simulink model "modelo_matematico"  (R2018b)
settings: Solver=ode4  StartTime=0.0  StopTime=t_f  FixedStep=fst  RelTol=1e-3  EnableMultiTasking=on
values from neighbouring files (symbols this model uses):
  a = plot(dado_t, dado_vd, '-', 'Color',[1.0,0.5,0.0], 'LineWidth', 4)    [Graficos.m]    (also in Trajetoria_OITO_8.m = 0.09)
  b = plot(dado_t, dado_vr, '-', 'Color',[0.0,0.0,0.0], 'LineWidth', 1)    [Graficos.m]    (also in Script_principal.m = 0.121)
  c_d = r_d/(2*b)    (= 0.120661157025)    [Script_principal.m]
  c_e = r_e/(2*b)    (= 0.121074380165)    [Script_principal.m]
  fD = 0.0069    [Script_principal.m]
  fD_v = var_fD*0.0069    (= 0.0069)    [Script_principal.m]
  fE = 0.0053    [Script_principal.m]
  fE_v = var_fE*0.0053    (= 0.0053)    [Script_principal.m]
  fst = 0.001    [Script_principal.m]
  I = 0.0903    [Script_principal.m]
  I_v = var_I*0.0903    (= 0.0903)    [Script_principal.m]
  Ir = 0.00094    [Script_principal.m]
  Ir_v = var_Ir*0.00094    (= 0.00094)    [Script_principal.m]
  k0 = 25    [Script_principal.m]
  k1 = 25    [Script_principal.m]
  KaD = 0.4713    [Script_principal.m]
  KaD_v = var_KaD*0.4713    (= 0.4713)    [Script_principal.m]
  KaE = 0.5046    [Script_principal.m]
  KaE_v = var_KaE*0.5046    (= 0.5046)    [Script_principal.m]
  KtD = KaD    (= 0.4713)    [Script_principal.m]
  KtD_v = var_KtD*KaD    (= 0.4713)    [Script_principal.m]
  KtE = KaE    (= 0.5046)    [Script_principal.m]
  KtE_v = var_KtE*KaE    (= 0.5046)    [Script_principal.m]
  L = 0.10    (= 0.1)    [Script_principal.m]
  m = 1.932    [Script_principal.m]
  m_v = var_m*1.932    (= 1.932)    [Script_principal.m]
  NL = 0    [Script_principal.m]
  npD = 0.0001    [Script_principal.m]
  npE = 0.0001    [Script_principal.m]
  r_d = 0.0292    [Script_principal.m]
  r_e = 0.0293    [Script_principal.m]
  RaD = 8.4507    [Script_principal.m]
  RaD_v = var_RaD*8.4507    (= 8.4507)    [Script_principal.m]
  RaE = 7.7177    [Script_principal.m]
  RaE_v = var_RaE*7.7177    (= 7.7177)    [Script_principal.m]
  T = 4    [Script_principal.m]
  t_f = t_i+dur_r+dur_8+dur_r    [Trajetoria_OITO_8.m]
  t_i = 0    [Trajetoria_OITO_8.m]
  t_i_1 = t_i+dur_r    (= 3.33333333333)    [Trajetoria_OITO_8.m]
  t_i_2 = t_i+dur_r+dur_8    [Trajetoria_OITO_8.m]
  v = 0.30    (= 0.3)    [Trajetoria_OITO_8.m]
  VaD_max = 14    [Script_principal.m]
  VaE_max = 14    [Script_principal.m]
  vel_ang_D = 4    [Script_principal.m]
  vel_ang_E = 4    [Script_principal.m]
  wx = v/raio_x    (= 0.3)    [Trajetoria_OITO_8.m]
  wy = v/raio_y    (= 0.6)    [Trajetoria_OITO_8.m]
  x0 = [x0_1; x0_2; x0_3; x0_4; x0_5; x0_6]    [Script_principal.m]
undefined symbols (not defined in the file or in its folder): dur_c, t_i_3, t_i_c, time_c, w
libraries: simulink x41, dspmtrx3 x8
settings Model: Creator=nenem  LastModifiedBy=nenem
settings OptimizationCC: LifeSpan=inf
settings DebuggingCC: SFUnexpectedBacktrackingDiag=warning  SFNoUnconditionalDefaultTransitionDiag=warning
settings SFSimCC: SimUseLocalCustomCode=off
settings RTWCC: RTWUseLocalCustomCode=off
settings CodeAppCC: StateflowObjectComments=on
settings GRTTargetCC: TargetLangStandard=C89/C90 (ANSI)  GeneratePreprocessorConditionals=Disable all
settings ConfigComp: CovMetricSettings=dw  CovHtmlReporting=on  CovSaveCumulativeToWorkspaceVar=on  CovSaveSingleToWorkspaceVar=on  CovExternalEMLEnable=off

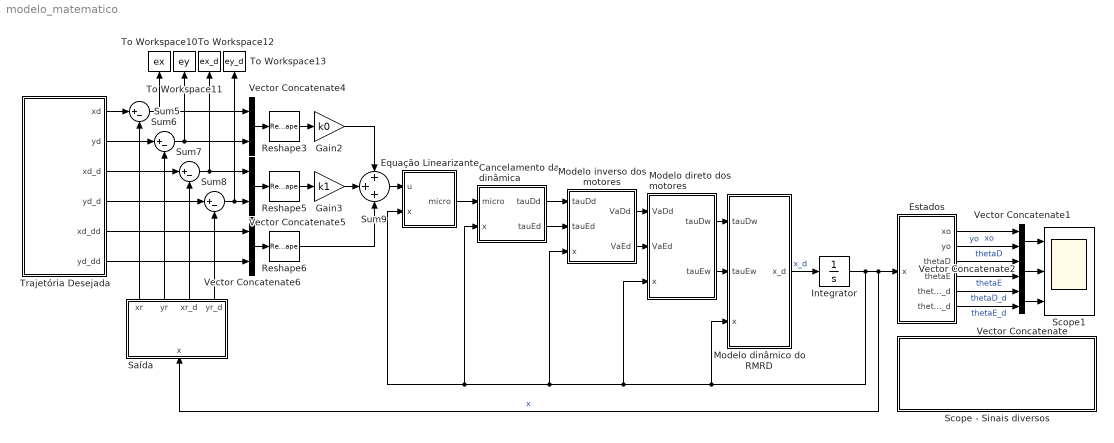
== system modelo_matematico ==
  Cancelamento da dinâmica : Subsystem
  Equação Linearizante : Subsystem
  Estados : Subsystem
  Gain2 : Gain  Gain=k0
  Gain3 : Gain  Gain=k1
  Integrator : Integrator  InitialCondition=x0
  Modelo dinâmico do RMRD : Subsystem
  Modelo direto dos motores : Subsystem
  Modelo inverso dos motores : Subsystem
  Reshape3 : Reshape  OutputDimensionality=Customize  OutputDimensions=[2,1]
  Reshape5 : Reshape  OutputDimensionality=Customize  OutputDimensions=[2,1]
  Reshape6 : Reshape  OutputDimensionality=Customize  OutputDimensions=[2,1]
  Saída : Subsystem
  Scope - Sinais diversos : Subsystem
  Scope1 : Scope  NumInputPorts=3
  Sum{5..8} (4 alike) : Sum  Inputs=|+-
  Sum9 : Sum  Inputs=+++
  To Workspace10 : ToWorkspace  VariableName=ex  SaveFormat=Structure With Time  SampleTime=-1
      settings: Save2DSignal=2-D array (concatenate along first dimension)
  To Workspace11 : ToWorkspace  VariableName=ey  SaveFormat=Structure With Time  SampleTime=-1
      settings: Save2DSignal=2-D array (concatenate along first dimension)
  To Workspace12 : ToWorkspace  VariableName=ex_d  SaveFormat=Structure With Time  SampleTime=-1
      settings: Save2DSignal=2-D array (concatenate along first dimension)
  To Workspace13 : ToWorkspace  VariableName=ey_d  SaveFormat=Structure With Time  SampleTime=-1
      settings: Save2DSignal=2-D array (concatenate along first dimension)
  Trajetória Desejada : Subsystem
  Vector Concatenate{,1..2,4..6} (6 alike) : Concatenate
  wires:
  Reshape6/1 -> Sum9/3
  Vector Concatenate6/1 -> Reshape6/1
  Reshape5/1 -> Gain3/1
  Sum7/1 -> Vector Concatenate5/1, To Workspace12/1
  Gain2/1 -> Sum9/1
  Equação Linearizante/1(micro) -> Cancelamento da dinâmica/1(micro)
  Sum8/1 -> Vector Concatenate5/2, To Workspace13/1
  Sum9/1 -> Equação Linearizante/1(u)
  Reshape3/1 -> Gain2/1
  Vector Concatenate5/1 -> Reshape5/1
  Vector Concatenate4/1 -> Reshape3/1
  Trajetória Desejada/3(xd_d) -> Sum7/1
  Trajetória Desejada/5(xd_dd) -> Vector Concatenate6/1
  Gain3/1 -> Sum9/2
  Trajetória Desejada/4(yd_d) -> Sum8/1
  Trajetória Desejada/2(yd) -> Sum6/1
  Trajetória Desejada/1(xd) -> Sum5/1
  Modelo dinâmico do RMRD/1(x_d) -> Integrator/1  "x_d"
  Integrator/1 -> Saída/1(x), Estados/1(x), Equação Linearizante/2(x), Cancelamento da dinâmica/2(x), Modelo inverso dos motores/3(x), Modelo direto dos motores/3(x), Modelo dinâmico do RMRD/3(x)  "x"
  Cancelamento da dinâmica/1(tauDd) -> Modelo inverso dos motores/1(tauDd)
  Cancelamento da dinâmica/2(tauEd) -> Modelo inverso dos motores/2(tauEd)
  Modelo direto dos motores/1(tauDw) -> Modelo dinâmico do RMRD/1(tauDw)
  Modelo direto dos motores/2(tauEw) -> Modelo dinâmico do RMRD/2(tauEw)
  Modelo inverso dos motores/2(VaEd) -> Modelo direto dos motores/2(VaEd)
  Modelo inverso dos motores/1(VaDd) -> Modelo direto dos motores/1(VaDd)
  Saída/1(xr) -> Sum5/2
  Saída/2(yr) -> Sum6/2
  Saída/3(xr_d) -> Sum7/2
  Saída/4(yr_d) -> Sum8/2
  Vector Concatenate1/1 -> Scope1/1
  Vector Concatenate2/1 -> Scope1/2
  Vector Concatenate/1 -> Scope1/3
  Estados/4(thetaE) -> Vector Concatenate2/2  "thetaE"
  Estados/1(xo) -> Vector Concatenate1/1  "xo"
  Estados/3(thetaD) -> Vector Concatenate2/1  "thetaD"
  Estados/2(yo) -> Vector Concatenate1/2  "yo"
  Estados/5(thetaD_d) -> Vector Concatenate/1  "thetaD_d"
  Estados/6(thetaE_d) -> Vector Concatenate/2  "thetaE_d"
  Trajetória Desejada/6(yd_dd) -> Vector Concatenate6/2
  Sum5/1 -> Vector Concatenate4/1, To Workspace10/1
  Sum6/1 -> Vector Concatenate4/2, To Workspace11/1

== system modelo_matematico/Cancelamento da dinâmica ==
  micro : Inport
  x : Inport  Port=2
  Constant1 : Constant  Value=[b r_d r_e c_d c_e Ir_v m_v I_v]
  Reshape7 : Reshape  OutputDimensionality=Customize  OutputDimensions=[1,8]
  To Workspace18 : ToWorkspace  VariableName=tauDd  SaveFormat=Structure With Time  SampleTime=-1
      settings: Save2DSignal=2-D array (concatenate along first dimension)
  To Workspace19 : ToWorkspace  VariableName=tauEd  SaveFormat=Structure With Time  SampleTime=-1
      settings: Save2DSignal=2-D array (concatenate along first dimension)
  Transformação da Entrada : MATLAB Function  TreatAsAtomicUnit=on
  tauDd : Outport
  tauEd : Outport  Port=2
  tag scope: tauDd=global, tauEd=global
  wires:
  micro/1 -> Transformação da Entrada/2(micro)
  Constant1/1 -> Reshape7/1
  Reshape7/1 -> Transformação da Entrada/1(cte)
  x/1 -> Transformação da Entrada/3(x)
  Transformação da Entrada/2(tauE) -> tauEd/1, To Workspace19/1, [tauEd]
  Transformação da Entrada/1(tauD) -> tauDd/1, To Workspace18/1, [tauDd]

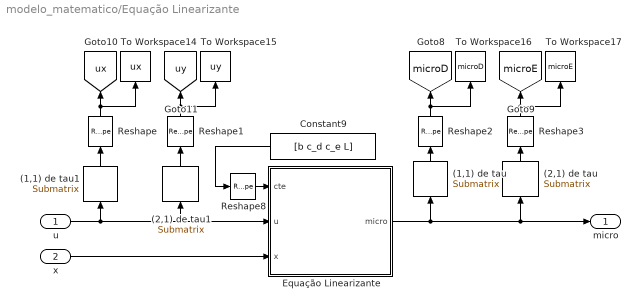
== system modelo_matematico/Equação Linearizante ==
  u : Inport
  x : Inport  Port=2
  (1,1) de tau : dspmtrx3/Submatrix  RowSpan=One row  RowStartMode=Index  RowStartIndex=1  RowEndMode=Last  RowEndIndex=1  ColSpan=One column  ColStartMode=Index  ColStartIndex=1  ColEndMode=Last  ColEndIndex=1
  (1,1) de tau1 : dspmtrx3/Submatrix  RowSpan=One row  RowStartMode=Index  RowStartIndex=1  RowEndMode=Last  RowEndIndex=1  ColSpan=One column  ColStartMode=Index  ColStartIndex=1  ColEndMode=Last  ColEndIndex=1
  (2,1) de tau : dspmtrx3/Submatrix  RowSpan=One row  RowStartMode=Index  RowStartIndex=2  RowEndMode=Last  RowEndIndex=1  ColSpan=One column  ColStartMode=Index  ColStartIndex=1  ColEndMode=Last  ColEndIndex=1
  (2,1) de tau1 : dspmtrx3/Submatrix  RowSpan=One row  RowStartMode=Index  RowStartIndex=2  RowEndMode=Last  RowEndIndex=1  ColSpan=One column  ColStartMode=Index  ColStartIndex=1  ColEndMode=Last  ColEndIndex=1
  Constant9 : Constant  Value=[b c_d c_e L]
  Equação Linearizante : MATLAB Function  TreatAsAtomicUnit=on
  Reshape{,1..3} (4 alike) : Reshape
  Reshape8 : Reshape  OutputDimensionality=Customize  OutputDimensions=[1,4]
  To Workspace14 : ToWorkspace  VariableName=ux  SaveFormat=Structure With Time  SampleTime=-1
      settings: Save2DSignal=2-D array (concatenate along first dimension)
  To Workspace15 : ToWorkspace  VariableName=uy  SaveFormat=Structure With Time  SampleTime=-1
      settings: Save2DSignal=2-D array (concatenate along first dimension)
  To Workspace16 : ToWorkspace  VariableName=microD  SaveFormat=Structure With Time  SampleTime=-1
      settings: Save2DSignal=2-D array (concatenate along first dimension)
  To Workspace17 : ToWorkspace  VariableName=microE  SaveFormat=Structure With Time  SampleTime=-1
      settings: Save2DSignal=2-D array (concatenate along first dimension)
  micro : Outport
  tag scope: microD=global, microE=global, ux=global, uy=global
  wires:
  Constant9/1 -> Reshape8/1
  Reshape8/1 -> Equação Linearizante/1(cte)
  x/1 -> Equação Linearizante/3(x)
  (2,1) de tau1/1 -> Reshape1/1
  (1,1) de tau1/1 -> Reshape/1
  u/1 -> (1,1) de tau1/1, (2,1) de tau1/1, Equação Linearizante/2(u)
  Reshape/1 -> To Workspace14/1, [ux]
  Reshape1/1 -> To Workspace15/1, [uy]
  Reshape3/1 -> To Workspace17/1, [microE]
  Reshape2/1 -> To Workspace16/1, [microD]
  (2,1) de tau/1 -> Reshape3/1
  Equação Linearizante/1(micro) -> micro/1, (2,1) de tau/1, (1,1) de tau/1
  (1,1) de tau/1 -> Reshape2/1

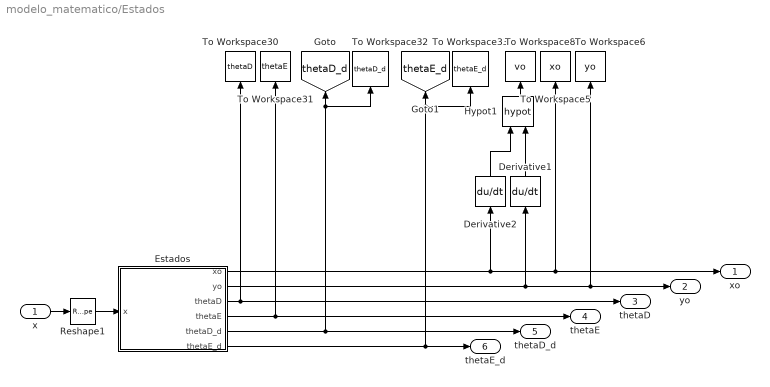
== system modelo_matematico/Estados ==
  x : Inport
  Derivative1 : Derivative
  Derivative2 : Derivative
  Estados : MATLAB Function  TreatAsAtomicUnit=on
  Hypot1 : Math  Operator=hypot  SaturateOnIntegerOverflow=on
  Reshape1 : Reshape  OutputDimensionality=Customize  OutputDimensions=[6,1]
  To Workspace30 : ToWorkspace  VariableName=thetaD  SaveFormat=Structure With Time  SampleTime=-1
      settings: Save2DSignal=2-D array (concatenate along first dimension)
  To Workspace31 : ToWorkspace  VariableName=thetaE  SaveFormat=Structure With Time  SampleTime=-1
      settings: Save2DSignal=2-D array (concatenate along first dimension)
  To Workspace32 : ToWorkspace  VariableName=thetaD_d  SaveFormat=Structure With Time  SampleTime=-1
      settings: Save2DSignal=2-D array (concatenate along first dimension)
  To Workspace33 : ToWorkspace  VariableName=thetaE_d  SaveFormat=Structure With Time  SampleTime=-1
      settings: Save2DSignal=2-D array (concatenate along first dimension)
  To Workspace5 : ToWorkspace  VariableName=xo  SaveFormat=Structure With Time  SampleTime=-1
      settings: Save2DSignal=2-D array (concatenate along first dimension)
  To Workspace6 : ToWorkspace  VariableName=yo  SaveFormat=Structure With Time  SampleTime=-1
      settings: Save2DSignal=2-D array (concatenate along first dimension)
  To Workspace8 : ToWorkspace  VariableName=vo  SaveFormat=Structure With Time  SampleTime=-1
      settings: Save2DSignal=2-D array (concatenate along first dimension)
  xo : Outport
  yo : Outport  Port=2
  thetaD : Outport  Port=3
  thetaE : Outport  Port=4
  thetaD_d : Outport  Port=5
  thetaE_d : Outport  Port=6
  tag scope: thetaD_d=global, thetaE_d=global
  wires:
  x/1 -> Reshape1/1
  Estados/5(thetaD_d) -> thetaD_d/1, To Workspace32/1, [thetaD_d]
  Estados/6(thetaE_d) -> thetaE_d/1, To Workspace33/1, [thetaE_d]
  Estados/1(xo) -> xo/1, To Workspace5/1, Derivative2/1
  Derivative2/1 -> Hypot1/1
  Estados/2(yo) -> yo/1, To Workspace6/1, Derivative1/1
  Derivative1/1 -> Hypot1/2
  Hypot1/1 -> To Workspace8/1
  Estados/3(thetaD) -> thetaD/1, To Workspace30/1
  Estados/4(thetaE) -> thetaE/1, To Workspace31/1
  Reshape1/1 -> Estados/1(x)

== system modelo_matematico/Modelo dinâmico do RMRD ==
  tauDw : Inport
  tauEw : Inport  Port=2
  x : Inport  Port=3
  Constant1 : Constant  Value=[b r_d r_e c_d c_e Ir m I]
  Manual Switch : ManualSwitch
  Modelo do WMR : MATLAB Function  TreatAsAtomicUnit=on
  Não idealidades : Subsystem  Commented=on
  Reshape2 : Reshape  OutputDimensionality=Customize  OutputDimensions=[1,8]
  Reshape3 : Reshape  OutputDimensionality=Customize  OutputDimensions=[6,1]
  x_d : Outport
  wires:
  tauEw/1 -> Modelo do WMR/3(tau_E)
  tauDw/1 -> Modelo do WMR/2(tau_D)
  Reshape2/1 -> Modelo do WMR/1(cte)
  Modelo do WMR/1(x_d) -> Reshape3/1  "x_d"
  x/1 -> Modelo do WMR/4(x)
  Reshape3/1 -> Manual Switch/1, Não idealidades/1(In)
  Manual Switch/1 -> x_d/1
  Constant1/1 -> Reshape2/1
  Não idealidades/1(Out) -> Manual Switch/2

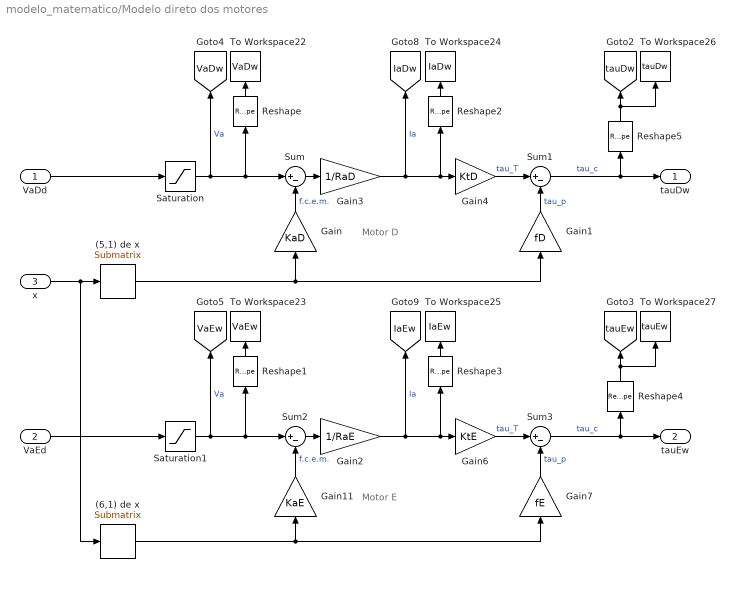
== system modelo_matematico/Modelo direto dos motores ==
  note: Motor D
  note: Motor E
  VaDd : Inport
  VaEd : Inport  Port=2
  x : Inport  Port=3
  (5,1) de x : dspmtrx3/Submatrix  RowSpan=One row  RowStartMode=Index  RowStartIndex=5  RowEndMode=Last  RowEndIndex=1  ColSpan=One column  ColStartMode=Index  ColStartIndex=1  ColEndMode=Last  ColEndIndex=1
  (6,1) de x : dspmtrx3/Submatrix  RowSpan=One row  RowStartMode=Index  RowStartIndex=6  RowEndMode=Last  RowEndIndex=1  ColSpan=One column  ColStartMode=Index  ColStartIndex=1  ColEndMode=Last  ColEndIndex=1
  Gain : Gain  Gain=KaD
  Gain1 : Gain  Gain=fD
  Gain11 : Gain  Gain=KaE
  Gain2 : Gain  Gain=1/RaE
  Gain3 : Gain  Gain=1/RaD
  Gain4 : Gain  Gain=KtD
  Gain6 : Gain  Gain=KtE
  Gain7 : Gain  Gain=fE
  Reshape{,1..5} (6 alike) : Reshape
  Saturation : Saturate  UpperLimit=VaD_max  LowerLimit=-VaD_max
  Saturation1 : Saturate  UpperLimit=VaE_max  LowerLimit=-VaE_max
  Sum{,1..3} (4 alike) : Sum  Inputs=|+-
  To Workspace22 : ToWorkspace  VariableName=VaDw  SaveFormat=Structure With Time  SampleTime=-1
      settings: Save2DSignal=2-D array (concatenate along first dimension)
  To Workspace23 : ToWorkspace  VariableName=VaEw  SaveFormat=Structure With Time  SampleTime=-1
      settings: Save2DSignal=2-D array (concatenate along first dimension)
  To Workspace24 : ToWorkspace  VariableName=IaDw  SaveFormat=Structure With Time  SampleTime=-1
      settings: Save2DSignal=2-D array (concatenate along first dimension)
  To Workspace25 : ToWorkspace  VariableName=IaEw  SaveFormat=Structure With Time  SampleTime=-1
      settings: Save2DSignal=2-D array (concatenate along first dimension)
  To Workspace26 : ToWorkspace  VariableName=tauDw  SaveFormat=Structure With Time  SampleTime=-1
      settings: Save2DSignal=2-D array (concatenate along first dimension)
  To Workspace27 : ToWorkspace  VariableName=tauEw  SaveFormat=Structure With Time  SampleTime=-1
      settings: Save2DSignal=2-D array (concatenate along first dimension)
  tauDw : Outport
  tauEw : Outport  Port=2
  tag scope: IaDw=global, IaEw=global, VaDw=global, VaEw=global, tauDw=global, tauEw=global
  wires:
  Gain7/1 -> Sum3/2  "tau_p"
  Gain2/1 -> Reshape3/1, Gain6/1, [IaEw]  "Ia"
  (6,1) de x/1 -> Gain11/1, Gain7/1
  Gain6/1 -> Sum3/1  "tau_T"
  (5,1) de x/1 -> Gain1/1, Gain/1
  Gain11/1 -> Sum2/2  "f.c.e.m."
  Gain1/1 -> Sum1/2  "tau_p"
  Sum2/1 -> Gain2/1
  Gain4/1 -> Sum1/1  "tau_T"
  Gain/1 -> Sum/2  "f.c.e.m."
  Gain3/1 -> Reshape2/1, Gain4/1, [IaDw]  "Ia"
  Sum/1 -> Gain3/1
  Sum1/1 -> Reshape5/1, tauDw/1  "tau_c"
  Sum3/1 -> Reshape4/1, tauEw/1  "tau_c"
  x/1 -> (5,1) de x/1, (6,1) de x/1
  Saturation/1 -> [VaDw], Reshape/1, Sum/1  "Va"
  Saturation1/1 -> [VaEw], Reshape1/1, Sum2/1  "Va"
  Reshape/1 -> To Workspace22/1
  Reshape1/1 -> To Workspace23/1
  Reshape2/1 -> To Workspace24/1
  Reshape3/1 -> To Workspace25/1
  VaDd/1 -> Saturation/1
  VaEd/1 -> Saturation1/1
  Reshape4/1 -> To Workspace27/1, [tauEw]
  Reshape5/1 -> To Workspace26/1, [tauDw]

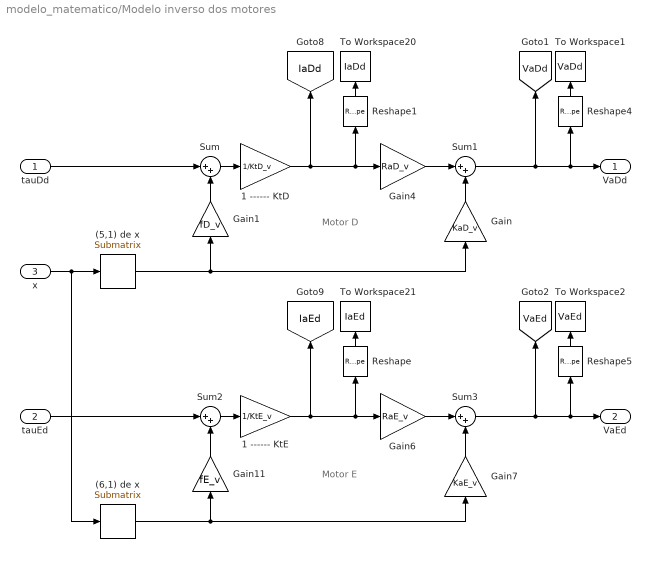
== system modelo_matematico/Modelo inverso dos motores ==
  note: Motor D
  note: Motor E
  tauDd : Inport
  tauEd : Inport  Port=2
  x : Inport  Port=3
  (5,1) de x : dspmtrx3/Submatrix  RowSpan=One row  RowStartMode=Index  RowStartIndex=5  RowEndMode=Last  RowEndIndex=1  ColSpan=One column  ColStartMode=Index  ColStartIndex=1  ColEndMode=Last  ColEndIndex=1
  (6,1) de x : dspmtrx3/Submatrix  RowSpan=One row  RowStartMode=Index  RowStartIndex=6  RowEndMode=Last  RowEndIndex=1  ColSpan=One column  ColStartMode=Index  ColStartIndex=1  ColEndMode=Last  ColEndIndex=1
  1 ------ KtD : Gain  Gain=1/KtD_v
  1 ------ KtE : Gain  Gain=1/KtE_v
  Gain : Gain  Gain=KaD_v
  Gain1 : Gain  Gain=fD_v
  Gain11 : Gain  Gain=fE_v
  Gain4 : Gain  Gain=RaD_v
  Gain6 : Gain  Gain=RaE_v
  Gain7 : Gain  Gain=KaE_v
  Reshape{,1,4..5} (4 alike) : Reshape
  Sum{,1..3} (4 alike) : Sum  Inputs=|++
  To Workspace1 : ToWorkspace  VariableName=VaDd  SaveFormat=Structure With Time  SampleTime=-1
      settings: Save2DSignal=2-D array (concatenate along first dimension)
  To Workspace2 : ToWorkspace  VariableName=VaEd  SaveFormat=Structure With Time  SampleTime=-1
      settings: Save2DSignal=2-D array (concatenate along first dimension)
  To Workspace20 : ToWorkspace  VariableName=IaDd  SaveFormat=Structure With Time  SampleTime=-1
      settings: Save2DSignal=2-D array (concatenate along first dimension)
  To Workspace21 : ToWorkspace  VariableName=IaEd  SaveFormat=Structure With Time  SampleTime=-1
      settings: Save2DSignal=2-D array (concatenate along first dimension)
  VaDd : Outport
  VaEd : Outport  Port=2
  tag scope: IaDd=global, IaEd=global, VaDd=global, VaEd=global
  wires:
  Gain7/1 -> Sum3/2
  1 ------ KtE/1 -> Reshape/1, Gain6/1, [IaEd]
  (6,1) de x/1 -> Gain11/1, Gain7/1
  Gain6/1 -> Sum3/1
  tauEd/1 -> Sum2/1
  (5,1) de x/1 -> Gain/1, Gain1/1
  Gain11/1 -> Sum2/2
  Gain/1 -> Sum1/2
  Sum2/1 -> 1 ------ KtE/1
  Gain4/1 -> Sum1/1
  Gain1/1 -> Sum/2
  1 ------ KtD/1 -> Reshape1/1, Gain4/1, [IaDd]
  Sum/1 -> 1 ------ KtD/1
  Sum1/1 -> [VaDd], VaDd/1, Reshape4/1
  Sum3/1 -> [VaEd], Reshape5/1, VaEd/1
  tauDd/1 -> Sum/1
  x/1 -> (6,1) de x/1, (5,1) de x/1
  Reshape/1 -> To Workspace21/1
  Reshape1/1 -> To Workspace20/1
  Reshape4/1 -> To Workspace1/1
  Reshape5/1 -> To Workspace2/1

== system modelo_matematico/Saída ==
  x : Inport
  Constant9 : Constant  Value=[b c_d c_e L]
  Hypot2 : Math  Operator=hypot  SaturateOnIntegerOverflow=on
  Reshape1 : Reshape  OutputDimensionality=Customize  OutputDimensions=[6,1]
  Reshape9 : Reshape  OutputDimensionality=Customize  OutputDimensions=[1,4]
  Saídas : MATLAB Function  TreatAsAtomicUnit=on
  To Workspace3 : ToWorkspace  VariableName=xr  SaveFormat=Structure With Time  SampleTime=-1
      settings: Save2DSignal=2-D array (concatenate along first dimension)
  To Workspace4 : ToWorkspace  VariableName=yr  SaveFormat=Structure With Time  SampleTime=-1
      settings: Save2DSignal=2-D array (concatenate along first dimension)
  To Workspace7 : ToWorkspace  VariableName=vr  SaveFormat=Structure With Time  SampleTime=-1
      settings: Save2DSignal=2-D array (concatenate along first dimension)
  xr : Outport
  yr : Outport  Port=2
  xr_d : Outport  Port=3
  yr_d : Outport  Port=4
  wires:
  Reshape9/1 -> Saídas/1(cte)
  Constant9/1 -> Reshape9/1
  x/1 -> Reshape1/1
  Saídas/3(xr_d) -> xr_d/1, Hypot2/1
  Saídas/4(yr_d) -> yr_d/1, Hypot2/2
  Saídas/1(xr) -> xr/1, To Workspace3/1
  Saídas/2(yr) -> yr/1, To Workspace4/1
  Hypot2/1 -> To Workspace7/1
  Reshape1/1 -> Saídas/2(x)

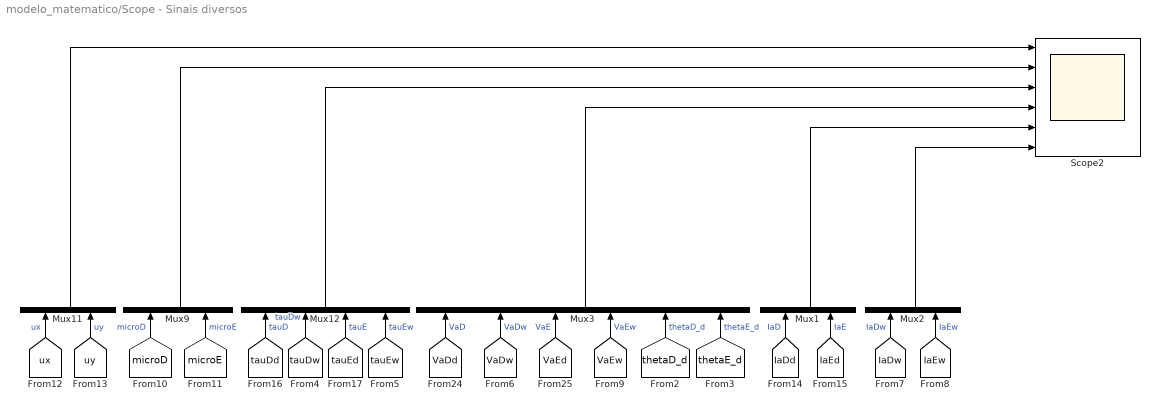
== system modelo_matematico/Scope - Sinais diversos ==
  Mux{1..2,9,11} (4 alike) : Mux  Inputs=2
  Mux12 : Mux
  Mux3 : Mux  Inputs=6
  Scope2 : Scope  NumInputPorts=6
  wires:
  [tauDd] -> Mux12/1  "tauD"
  [VaEw] -> Mux3/4  "VaEw"
  [IaEd] -> Mux1/2  "IaE"
  [ux] -> Mux11/1  "ux"
  [VaEd] -> Mux3/3  "VaE"
  [IaDd] -> Mux1/1  "IaD"
  [VaDw] -> Mux3/2  "VaDw"
  [tauEd] -> Mux12/3  "tauE"
  Mux12/1 -> Scope2/3
  [uy] -> Mux11/2  "uy"
  Mux3/1 -> Scope2/4
  [microD] -> Mux9/1  "microD"
  [microE] -> Mux9/2  "microE"
  [VaDd] -> Mux3/1  "VaD"
  Mux11/1 -> Scope2/1
  Mux9/1 -> Scope2/2
  Mux1/1 -> Scope2/5
  Mux2/1 -> Scope2/6
  [tauDw] -> Mux12/2  "tauDw"
  [tauEw] -> Mux12/4  "tauEw"
  [thetaD_d] -> Mux3/5  "thetaD_d"
  [thetaE_d] -> Mux3/6  "thetaE_d"
  [IaEw] -> Mux2/2  "IaEw"
  [IaDw] -> Mux2/1  "IaDw"

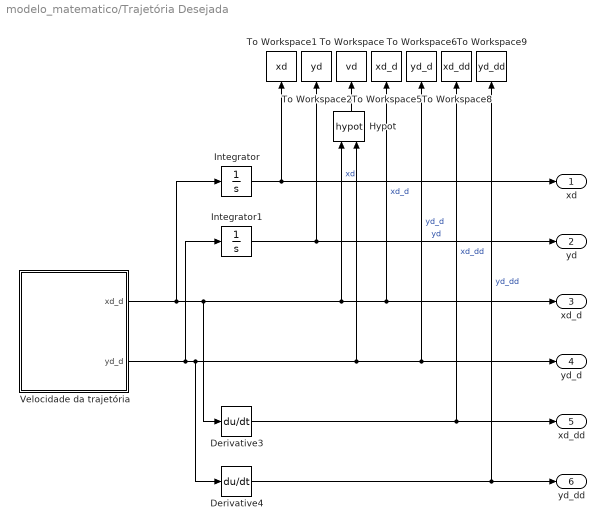
== system modelo_matematico/Trajetória Desejada ==
  Derivative3 : Derivative
  Derivative4 : Derivative
  Hypot : Math  Operator=hypot  OutputSignalType=real  SaturateOnIntegerOverflow=on
  Integrator : Integrator
  Integrator1 : Integrator
  To Workspace : ToWorkspace  VariableName=vd  SaveFormat=Structure With Time  SampleTime=-1
      settings: Save2DSignal=2-D array (concatenate along first dimension)
  To Workspace1 : ToWorkspace  VariableName=xd  SaveFormat=Structure With Time  SampleTime=-1
      settings: Save2DSignal=2-D array (concatenate along first dimension)
  To Workspace2 : ToWorkspace  VariableName=yd  SaveFormat=Structure With Time  SampleTime=-1
      settings: Save2DSignal=2-D array (concatenate along first dimension)
  To Workspace5 : ToWorkspace  VariableName=xd_d  SaveFormat=Structure With Time  SampleTime=-1
      settings: Save2DSignal=2-D array (concatenate along first dimension)
  To Workspace6 : ToWorkspace  VariableName=yd_d  SaveFormat=Structure With Time  SampleTime=-1
      settings: Save2DSignal=2-D array (concatenate along first dimension)
  To Workspace8 : ToWorkspace  VariableName=xd_dd  SaveFormat=Structure With Time  SampleTime=-1
      settings: Save2DSignal=2-D array (concatenate along first dimension)
  To Workspace9 : ToWorkspace  VariableName=yd_dd  SaveFormat=Structure With Time  SampleTime=-1
      settings: Save2DSignal=2-D array (concatenate along first dimension)
  Velocidade da trajetória : Subsystem
  xd : Outport
  yd : Outport  Port=2
  xd_d : Outport  Port=3
  yd_d : Outport  Port=4
  xd_dd : Outport  Port=5
  yd_dd : Outport  Port=6
  wires:
  Derivative3/1 -> xd_dd/1, To Workspace8/1  "xd_dd"
  Derivative4/1 -> yd_dd/1, To Workspace9/1  "yd_dd"
  Integrator/1 -> xd/1, To Workspace1/1  "xd"
  Integrator1/1 -> yd/1, To Workspace2/1  "yd"
  Hypot/1 -> To Workspace/1
  Velocidade da trajetória/1(xd_d) -> Integrator/1, Derivative3/1, xd_d/1, To Workspace5/1, Hypot/1  "xd_d"
  Velocidade da trajetória/2(yd_d) -> Integrator1/1, yd_d/1, To Workspace6/1, Hypot/2, Derivative4/1  "yd_d"

== system modelo_matematico/Modelo dinâmico do RMRD/Não idealidades ==
  In : Inport
  Não idealidades : Subsystem
  demux : MATLAB Function  TreatAsAtomicUnit=on
  mux : MATLAB Function  TreatAsAtomicUnit=on
  Out : Outport
  wires:
  In/1 -> demux/1(x)
  Não idealidades/1(OutD) -> mux/5(x5_d)
  Não idealidades/2(OutE) -> mux/6(x6_d)
  mux/1(x) -> Out/1
  demux/5(x5_d) -> Não idealidades/1(InD)
  demux/6(x6_d) -> Não idealidades/2(InE)
  demux/4(x4_d) -> mux/4(x4_d)
  demux/2(x2_d) -> mux/2(x2_d)
  demux/1(x1_d) -> mux/1(x1_d)
  demux/3(x3_d) -> mux/3(x3_d)

== system modelo_matematico/Trajetória Desejada/Velocidade da trajetória ==
  0 : Subsystem  Commented=on
  0 c/ RAMPA : Subsystem  Commented=on
  180 c/ RAMPA : Subsystem  Commented=on
  8 : Subsystem
  "90 " : Subsystem  Commented=on
  90 c/ RAMPA : Subsystem  Commented=on
  Constant : Constant  Value=T
  Multiport Switch : MultiPortSwitch  Inputs=4
  Multiport Switch1 : MultiPortSwitch  Inputs=4
  Reta c/ RAMPA : Subsystem  Commented=on
  xd_d : Outport
  yd_d : Outport  Port=2
  wires:
  0 c/ RAMPA/2(yd_d) -> Multiport Switch1/2  "yd_d"
  90 c/ RAMPA/2(yd_d) -> Multiport Switch1/3  "yd_d"
  90 c/ RAMPA/1(xd_d) -> Multiport Switch/3  "xd_d"
  0 c/ RAMPA/1(xd_d) -> Multiport Switch/2  "xd_d"
  Constant/1 -> Multiport Switch/1, Multiport Switch1/1
  Multiport Switch/1 -> xd_d/1  "xd_d"
  Multiport Switch1/1 -> yd_d/1  "yd_d"
  8/2(yd_d) -> Multiport Switch1/5  "yd_d"
  180 c/ RAMPA/2(yd_d) -> Multiport Switch1/4  "yd_d"
  180 c/ RAMPA/1(xd_d) -> Multiport Switch/4  "xd_d"
  8/1(xd_d) -> Multiport Switch/5

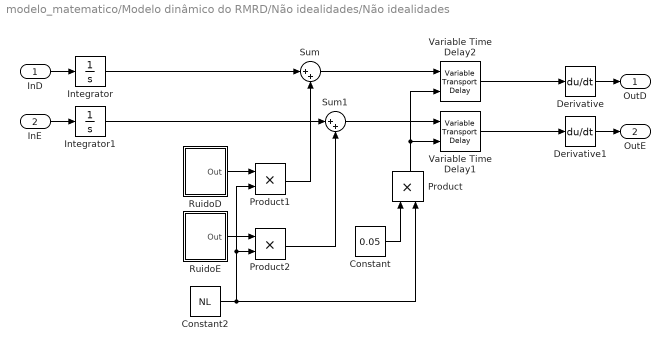
== system modelo_matematico/Modelo dinâmico do RMRD/Não idealidades/Não idealidades ==
  InD : Inport
  InE : Inport  Port=2
  Constant : Constant  Value=0.05
  Constant2 : Constant  Value=NL
  Derivative : Derivative
  Derivative1 : Derivative
  Integrator : Integrator
  Integrator1 : Integrator
  Product : Product
  Product1 : Product
  Product2 : Product
  RuidoD : Subsystem
  RuidoE : Subsystem
  Sum : Sum  Inputs=|++
  Sum1 : Sum  Inputs=|++
  Variable Time Delay1 : VariableTransportDelay  MaximumDelay=10
  Variable Time Delay2 : VariableTransportDelay  MaximumDelay=10
  OutD : Outport
  OutE : Outport  Port=2
  wires:
  RuidoE/1(Out) -> Product2/1
  Integrator/1 -> Sum/1
  Constant2/1 -> Product1/2, Product2/2, Product/2
  Integrator1/1 -> Sum1/1
  Variable Time Delay1/1 -> Derivative1/1
  Product/1 -> Variable Time Delay1/2, Variable Time Delay2/2
  Product2/1 -> Sum1/2
  Sum1/1 -> Variable Time Delay1/1
  Constant/1 -> Product/1
  Product1/1 -> Sum/2
  RuidoD/1(Out) -> Product1/1
  Sum/1 -> Variable Time Delay2/1
  Variable Time Delay2/1 -> Derivative/1
  Derivative1/1 -> OutE/1
  Derivative/1 -> OutD/1
  InE/1 -> Integrator1/1
  InD/1 -> Integrator/1

== system modelo_matematico/Trajetória Desejada/Velocidade da trajetória/0 ==
  Gain : Gain  Gain=w
  Gain1 : Gain  Gain=v
  Gain2 : Gain  Gain=w
  Gain3 : Gain  Gain=v
  Gain4 : Gain  Gain=-1
  Ramp18 : simulink/Sources/Ramp  slope=1  start=t_i  InitialOutput=0
  Ramp19 : simulink/Sources/Ramp  slope=-1  start=t_i  InitialOutput=0
  Trigonometric Function : Trigonometry
  Trigonometric Function1 : Trigonometry  Operator=cos
  xd_d : Outport
  yd_d : Outport  Port=2
  wires:
  Gain4/1 -> Gain1/1
  Ramp18/1 -> Gain/1
  Gain/1 -> Trigonometric Function/1
  Trigonometric Function1/1 -> Gain3/1
  Gain2/1 -> Trigonometric Function1/1
  Ramp19/1 -> Gain2/1
  Gain1/1 -> xd_d/1
  Gain3/1 -> yd_d/1
  Trigonometric Function/1 -> Gain4/1

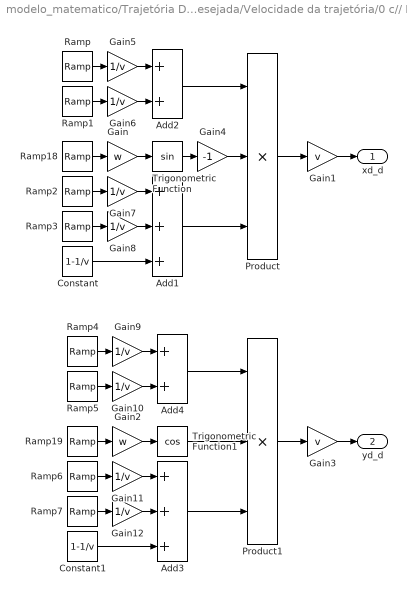
== system modelo_matematico/Trajetória Desejada/Velocidade da trajetória/0 c// RAMPA ==
  Add1 : Sum  Inputs=3
  Add2 : Sum  Inputs=2
  Add3 : Sum  Inputs=3
  Add4 : Sum  Inputs=2
  Constant : Constant  Value=1-1/v
  Constant1 : Constant  Value=1-1/v
  Gain : Gain  Gain=w
  Gain1 : Gain  Gain=v
  Gain{5..12} (8 alike) : Gain  Gain=1/v
  Gain2 : Gain  Gain=w
  Gain3 : Gain  Gain=v
  Gain4 : Gain  Gain=-1
  Product : Product  Inputs=3
  Product1 : Product  Inputs=3
  Ramp : simulink/Sources/Ramp  slope=a  start=t_i  InitialOutput=0
  Ramp1 : simulink/Sources/Ramp  slope=-a  start=t_1  InitialOutput=0
  Ramp18 : simulink/Sources/Ramp  slope=1  start=t_i  InitialOutput=0
  Ramp19 : simulink/Sources/Ramp  slope=1  start=t_i  InitialOutput=0
  Ramp2 : simulink/Sources/Ramp  slope=-a  start=t_2  InitialOutput=1
  Ramp3 : simulink/Sources/Ramp  slope=a  start=t_f  InitialOutput=0
  Ramp4 : simulink/Sources/Ramp  slope=a  start=t_i  InitialOutput=0
  Ramp5 : simulink/Sources/Ramp  slope=-a  start=t_1  InitialOutput=0
  Ramp6 : simulink/Sources/Ramp  slope=-a  start=t_2  InitialOutput=1
  Ramp7 : simulink/Sources/Ramp  slope=a  start=t_f  InitialOutput=0
  Trigonometric Function : Trigonometry
  Trigonometric Function1 : Trigonometry  Operator=cos
  xd_d : Outport
  yd_d : Outport  Port=2
  wires:
  Product/1 -> Gain1/1
  Ramp18/1 -> Gain/1
  Gain/1 -> Trigonometric Function/1
  Gain2/1 -> Trigonometric Function1/1
  Ramp19/1 -> Gain2/1
  Gain1/1 -> xd_d/1
  Gain3/1 -> yd_d/1
  Trigonometric Function/1 -> Gain4/1
  Ramp/1 -> Gain5/1
  Ramp1/1 -> Gain6/1
  Gain5/1 -> Add2/1
  Gain6/1 -> Add2/2
  Add2/1 -> Product/1
  Gain4/1 -> Product/2
  Product1/1 -> Gain3/1
  Trigonometric Function1/1 -> Product1/2
  Ramp2/1 -> Gain7/1
  Gain7/1 -> Add1/1
  Ramp3/1 -> Gain8/1
  Gain8/1 -> Add1/2
  Add1/1 -> Product/3
  Constant/1 -> Add1/3
  Ramp6/1 -> Gain11/1
  Add3/1 -> Product1/3
  Constant1/1 -> Add3/3
  Gain12/1 -> Add3/2
  Gain9/1 -> Add4/1
  Add4/1 -> Product1/1
  Gain11/1 -> Add3/1
  Ramp4/1 -> Gain9/1
  Ramp7/1 -> Gain12/1
  Gain10/1 -> Add4/2
  Ramp5/1 -> Gain10/1

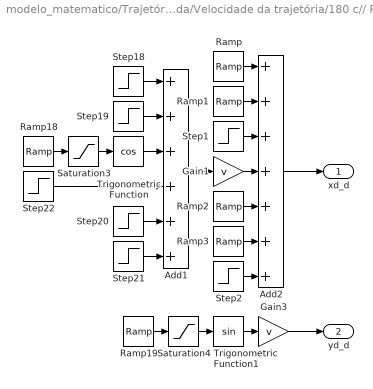
== system modelo_matematico/Trajetória Desejada/Velocidade da trajetória/180 c// RAMPA ==
  Add1 : Sum  Inputs=++++++
  Add2 : Sum  Inputs=+++++++
  Gain1 : Gain  Gain=v
  Gain3 : Gain  Gain=v
  Ramp : simulink/Sources/Ramp  slope=a  start=t_i  InitialOutput=0
  Ramp1 : simulink/Sources/Ramp  slope=-a  start=t_i_1  InitialOutput=0
  Ramp18 : simulink/Sources/Ramp  slope=pi/dur_c  start=t_i_c  InitialOutput=0
  Ramp19 : simulink/Sources/Ramp  slope=pi/dur_c  start=t_i_c  InitialOutput=0
  Ramp2 : simulink/Sources/Ramp  slope=a  start=t_i_3  InitialOutput=0
  Ramp3 : simulink/Sources/Ramp  slope=-a  start=t_f  InitialOutput=0
  Saturation3 : Saturate  UpperLimit=pi  LowerLimit=0
  Saturation4 : Saturate  UpperLimit=pi  LowerLimit=0
  Step1 : Step  Time=t_i_1  After=-v  SampleTime=0
  Step18 : Step  Time=t_i_1  SampleTime=0
  Step19 : Step  Time=t_i_c  After=-1  SampleTime=0
  Step2 : Step  Time=t_i_3  After=-v  SampleTime=0
  Step20 : Step  Time=t_i_3  SampleTime=0
  Step21 : Step  Time=t_f  After=-1  SampleTime=0
  Step22 : Step  Time=t_i_c  Before=-1  After=0  SampleTime=0
  Trigonometric Function : Trigonometry  Operator=cos
  Trigonometric Function1 : Trigonometry
  xd_d : Outport
  yd_d : Outport  Port=2
  wires:
  Add1/1 -> Gain1/1
  Ramp18/1 -> Saturation3/1
  Saturation3/1 -> Trigonometric Function/1
  Saturation4/1 -> Trigonometric Function1/1
  Ramp19/1 -> Saturation4/1
  Step18/1 -> Add1/1
  Step19/1 -> Add1/2
  Trigonometric Function/1 -> Add1/3
  Step22/1 -> Add1/4
  Add2/1 -> xd_d/1
  Ramp/1 -> Add2/1
  Ramp1/1 -> Add2/2
  Step1/1 -> Add2/3
  Gain1/1 -> Add2/4
  Gain3/1 -> yd_d/1
  Ramp2/1 -> Add2/5
  Ramp3/1 -> Add2/6
  Step20/1 -> Add1/5
  Step21/1 -> Add1/6
  Step2/1 -> Add2/7
  Trigonometric Function1/1 -> Gain3/1

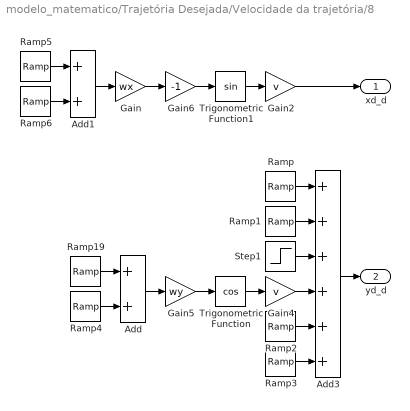
== system modelo_matematico/Trajetória Desejada/Velocidade da trajetória/8 ==
  Add : Sum
  Add1 : Sum
  Add3 : Sum  Inputs=++++++
  Gain : Gain  Gain=wx
  Gain2 : Gain  Gain=v
  Gain4 : Gain  Gain=v
  Gain5 : Gain  Gain=wy
  Gain6 : Gain  Gain=-1
  Ramp : simulink/Sources/Ramp  slope=a  start=t_i  InitialOutput=0
  Ramp1 : simulink/Sources/Ramp  slope=-a  start=t_i_1  InitialOutput=0
  Ramp19 : simulink/Sources/Ramp  slope=1  start=t_i_1  InitialOutput=0
  Ramp2 : simulink/Sources/Ramp  slope=-a  start=t_i_2  InitialOutput=0
  Ramp3 : simulink/Sources/Ramp  slope=a  start=t_f  InitialOutput=0
  Ramp4 : simulink/Sources/Ramp  slope=-1  start=t_i_2  InitialOutput=0
  Ramp5 : simulink/Sources/Ramp  slope=1  start=t_i_1  InitialOutput=0
  Ramp6 : simulink/Sources/Ramp  slope=-1  start=t_i_2  InitialOutput=0
  Step1 : Step  Time=t_i  After=-v  SampleTime=0
  Trigonometric Function : Trigonometry  Operator=cos
  Trigonometric Function1 : Trigonometry
  xd_d : Outport
  yd_d : Outport  Port=2
  wires:
  Add1/1 -> Gain/1
  Trigonometric Function/1 -> Gain4/1
  Trigonometric Function1/1 -> Gain2/1
  Add3/1 -> yd_d/1
  Gain/1 -> Gain6/1
  Gain5/1 -> Trigonometric Function/1
  Gain6/1 -> Trigonometric Function1/1
  Gain4/1 -> Add3/4
  Ramp2/1 -> Add3/5
  Ramp3/1 -> Add3/6
  Ramp1/1 -> Add3/2
  Ramp/1 -> Add3/1
  Step1/1 -> Add3/3
  Ramp19/1 -> Add/1
  Add/1 -> Gain5/1
  Ramp4/1 -> Add/2
  Ramp6/1 -> Add1/2
  Ramp5/1 -> Add1/1
  Gain2/1 -> xd_d/1

== system modelo_matematico/Trajetória Desejada/Velocidade da trajetória/90  ==
  Add7 : Sum  Inputs=++++
  Add8 : Sum  Inputs=++++
  Gain1 : Gain  Gain=v
  Gain3 : Gain  Gain=v
  Ramp18 : simulink/Sources/Ramp  slope=(pi/2)/time_c  start=t_i_c  InitialOutput=0
  Ramp19 : simulink/Sources/Ramp  slope=(pi/2)/time_c  start=t_i_c  InitialOutput=0
  Saturation3 : Saturate  UpperLimit=pi/2  LowerLimit=0
  Saturation4 : Saturate  UpperLimit=pi/2  LowerLimit=0
  Step18 : Step  Time=t_i  SampleTime=0
  Step19 : Step  Time=t_i_c  After=-1  SampleTime=0
  Step20 : Step  Time=t_i_2  SampleTime=0
  Step21 : Step  Time=t_f  After=-1  SampleTime=0
  Step22 : Step  Time=t_i_c  Before=-1  After=0  SampleTime=0
  Step23 : Step  Time=t_i_2  After=-1  SampleTime=0
  Trigonometric Function : Trigonometry  Operator=cos
  Trigonometric Function1 : Trigonometry
  xd_d : Outport
  yd_d : Outport  Port=2
  wires:
  Add7/1 -> Gain1/1
  Ramp18/1 -> Saturation3/1
  Step21/1 -> Add8/4
  Saturation3/1 -> Trigonometric Function/1
  Add8/1 -> Gain3/1
  Step20/1 -> Add8/3
  Trigonometric Function1/1 -> Add8/1
  Saturation4/1 -> Trigonometric Function1/1
  Ramp19/1 -> Saturation4/1
  Step23/1 -> Add8/2
  Gain1/1 -> xd_d/1
  Gain3/1 -> yd_d/1
  Step22/1 -> Add7/4
  Trigonometric Function/1 -> Add7/3
  Step19/1 -> Add7/2
  Step18/1 -> Add7/1

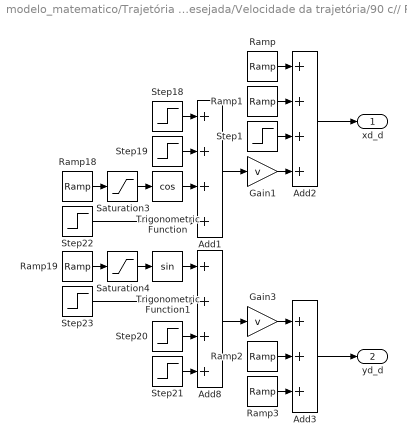
== system modelo_matematico/Trajetória Desejada/Velocidade da trajetória/90 c// RAMPA ==
  Add1 : Sum  Inputs=++++
  Add2 : Sum  Inputs=++++
  Add3 : Sum  Inputs=+++
  Add8 : Sum  Inputs=++++
  Gain1 : Gain  Gain=v
  Gain3 : Gain  Gain=v
  Ramp : simulink/Sources/Ramp  slope=a  start=t_i  InitialOutput=0
  Ramp1 : simulink/Sources/Ramp  slope=-a  start=t_i_1  InitialOutput=0
  Ramp18 : simulink/Sources/Ramp  slope=(pi/2)/dur_c  start=t_i_c  InitialOutput=0
  Ramp19 : simulink/Sources/Ramp  slope=(pi/2)/dur_c  start=t_i_c  InitialOutput=0
  Ramp2 : simulink/Sources/Ramp  slope=-a  start=t_i_3  InitialOutput=0
  Ramp3 : simulink/Sources/Ramp  slope=a  start=t_f  InitialOutput=0
  Saturation3 : Saturate  UpperLimit=pi/2  LowerLimit=0
  Saturation4 : Saturate  UpperLimit=pi/2  LowerLimit=0
  Step1 : Step  Time=t_i_1  After=-v  SampleTime=0
  Step18 : Step  Time=t_i_1  SampleTime=0
  Step19 : Step  Time=t_i_c  After=-1  SampleTime=0
  Step20 : Step  Time=t_i_2  SampleTime=0
  Step21 : Step  Time=t_f  After=-1  SampleTime=0
  Step22 : Step  Time=t_i_c  Before=-1  After=0  SampleTime=0
  Step23 : Step  Time=t_i_2  After=-1  SampleTime=0
  Trigonometric Function : Trigonometry  Operator=cos
  Trigonometric Function1 : Trigonometry
  xd_d : Outport
  yd_d : Outport  Port=2
  wires:
  Add1/1 -> Gain1/1
  Ramp18/1 -> Saturation3/1
  Step21/1 -> Add8/4
  Saturation3/1 -> Trigonometric Function/1
  Add8/1 -> Gain3/1
  Step20/1 -> Add8/3
  Trigonometric Function1/1 -> Add8/1
  Saturation4/1 -> Trigonometric Function1/1
  Ramp19/1 -> Saturation4/1
  Step23/1 -> Add8/2
  Step18/1 -> Add1/1
  Step19/1 -> Add1/2
  Trigonometric Function/1 -> Add1/3
  Step22/1 -> Add1/4
  Add2/1 -> xd_d/1
  Ramp/1 -> Add2/1
  Ramp1/1 -> Add2/2
  Step1/1 -> Add2/3
  Gain1/1 -> Add2/4
  Gain3/1 -> Add3/1
  Add3/1 -> yd_d/1
  Ramp2/1 -> Add3/2
  Ramp3/1 -> Add3/3

== system modelo_matematico/Trajetória Desejada/Velocidade da trajetória/Reta c// RAMPA ==
  Add1 : Sum
  Add2 : Sum  Inputs=++++++
  Constant : Constant  Value=0
  Gain1 : Gain  Gain=v
  Ramp : simulink/Sources/Ramp  slope=a  start=t_i  InitialOutput=0
  Ramp1 : simulink/Sources/Ramp  slope=-a  start=t_i_1  InitialOutput=0
  Ramp2 : simulink/Sources/Ramp  slope=-a  start=t_i_2  InitialOutput=0
  Step1 : Step  Time=t_i_1  After=-v  SampleTime=0
  Step18 : Step  Time=t_i_1  SampleTime=0
  Step19 : Step  Time=t_i_2  After=-1  SampleTime=0
  Step2 : Step  Time=t_i_2  After=v  SampleTime=0
  xd_d : Outport
  yd_d : Outport  Port=2
  wires:
  Add1/1 -> Gain1/1
  Step18/1 -> Add1/1
  Step19/1 -> Add1/2
  Add2/1 -> xd_d/1
  Ramp/1 -> Add2/1
  Ramp1/1 -> Add2/2
  Step1/1 -> Add2/3
  Gain1/1 -> Add2/4
  Ramp2/1 -> Add2/5
  Step2/1 -> Add2/6
  Constant/1 -> yd_d/1

== system modelo_matematico/Modelo dinâmico do RMRD/Não idealidades/Não idealidades/RuidoD ==
  Band-Limited White Noise : simulink/Sources/Band-Limited White Noise  Cov=[npD]  Ts=fst  seed=[23341]
  Gain : Gain  Gain=2
  Ramp39 : simulink/Sources/Ramp  slope=vel_ang_D*2*pi  start=0  InitialOutput=0
  Sum13 : Sum
  Trigonometric Function4 : Trigonometry
  Out : Outport
  wires:
  Band-Limited White Noise/1 -> Sum13/1
  Trigonometric Function4/1 -> Gain/1
  Ramp39/1 -> Trigonometric Function4/1
  Sum13/1 -> Out/1
  Gain/1 -> Sum13/2

== system modelo_matematico/Modelo dinâmico do RMRD/Não idealidades/Não idealidades/RuidoE ==
  Band-Limited White Noise : simulink/Sources/Band-Limited White Noise  Cov=[npE]  Ts=fst  seed=[23341]
  Gain : Gain  Gain=2
  Ramp39 : simulink/Sources/Ramp  slope=vel_ang_E*2*pi  start=0  InitialOutput=0
  Sum13 : Sum
  Trigonometric Function4 : Trigonometry  Operator=cos
  Out : Outport
  wires:
  Band-Limited White Noise/1 -> Sum13/1
  Trigonometric Function4/1 -> Gain/1
  Ramp39/1 -> Trigonometric Function4/1
  Sum13/1 -> Out/1
  Gain/1 -> Sum13/2

== matlab function modelo_matematico/Estados/Estados ==
  data: xo output; yo output; x input; thetaD output; thetaE output; thetaD_d output; thetaE_d output
function [xo, yo, thetaD, thetaE, thetaD_d, thetaE_d] = fcn(x)

%#codegen
%--------------------------------------------------------------------------
xo     = x(1,1);
yo     = x(2,1);
thetaD   = x(3,1);
thetaE   = x(4,1);
thetaD_d = x(5,1);
thetaE_d = x(6,1);

== matlab function modelo_matematico/Modelo dinâmico do RMRD/Não idealidades/demux ==
  data: x1_d output; x2_d output; x input; x3_d output; x4_d output; x5_d output; x6_d output
function [x1_d, x2_d, x3_d, x4_d, x5_d, x6_d] = fcn(x)

%#codegen
%--------------------------------------------------------------------------
x1_d = x(1,1);
x2_d = x(2,1);
x3_d = x(3,1);
x4_d = x(4,1);
x5_d = x(5,1);
x6_d = x(6,1);

== matlab function modelo_matematico/Modelo dinâmico do RMRD/Modelo do WMR ==
  data: cte input; tau_D input; tau_E input; x input; x_d output
function x_d = fcn(cte, tau_D, tau_E, x)
%#codegen
% Parametros de simulação--------------------------------------------------
% eta = η;

b   = cte(1,1);
r_d = cte(1,2);
r_e = cte(1,3);
c_d = cte(1,4);
c_e = cte(1,5);
Ir  = cte(1,6);
m   = cte(1,7);
I   = cte(1,8);

%--------------------------------------------------------------------------
thetaD_d = x(5,1);
thetaE_d = x(6,1);
phi      = c_d*x(3,1)-c_e*x(4,1);

%--------------------------------------------------------------------------
S = [ c_d*b*cos(phi) , c_e*b*cos(phi) ;
      c_d*b*sin(phi) , c_e*b*sin(phi) ;
            1        ,       0        ;
            0        ,       1        ];
               
S_d = [ -(r_d^2/4*b)*sin(phi)*thetaD_d + (r_d*r_e/4*b)*sin(phi)*thetaE_d , -(r_d*r_e/4*b)*sin(phi)*thetaD_d + (r_e^2/4*b)*sin(phi)*thetaE_d;
         (r_d^2/4*b)*cos(phi)*thetaD_d - (r_d*r_e/4*b)*cos(phi)*thetaE_d ,  (r_d*r_e/4*b)*cos(phi)*thetaD_d - (r_e^2/4*b)*cos(phi)*thetaE_d;
                                       0                                 ,                                  0                              ;
                                       0                                 ,                                  0                              ];
                        
M = [ m , 0 ,       0    ,       0    ;
      0 , m ,       0    ,       0    ;
      0 , 0 , Ir+I*c_d^2 ,   -I*c_e^2 ;
      0 , 0 ,   -I*c_d^2 , Ir+I*c_e^2 ];
            
eta = [thetaD_d;
       thetaE_d];
   
f2 = -(S'*M*S)^-1*(S'*M*S_d*eta);

%--------------------------------------------------------------------------
tau = [tau_D;
       tau_E];
   
x_d = [ S*eta ; f2 ] + [ 0 0 ; 0 0 ; 0 0 ; 0 0 ; (S'*M*S)^-1 ]*tau;

== matlab function modelo_matematico/Modelo dinâmico do RMRD/Não idealidades/mux ==
  data: x output; x1_d input; x2_d input; x3_d input; x4_d input; x5_d input; x6_d input
function x = fcn(x1_d, x2_d, x3_d, x4_d, x5_d, x6_d)

%#codegen
%--------------------------------------------------------------------------
x = [x1_d; x2_d; x3_d; x4_d; x5_d; x6_d];

== matlab function modelo_matematico/Equação Linearizante/Equação Linearizante ==
  data: cte input; u input; x input; micro output
function micro = fcn(cte, u, x)
%#codegen
% Parametros de simulação--------------------------------------------------
% micro = µ;
% eta = η;

b   = cte(1,1);
c_d = cte(1,2);
c_e = cte(1,3);
L   = cte(1,4);

%--------------------------------------------------------------------------
thetaD_d = x(5,1);
thetaE_d = x(6,1);
phi      = c_d*x(3,1)-c_e*x(4,1);

%--------------------------------------------------------------------------
LgLfh = [c_d*b*cos(phi)-c_d*L*sin(phi) c_e*b*cos(phi)+c_e*L*sin(phi);
         c_d*b*sin(phi)+c_d*L*cos(phi) c_e*b*sin(phi)-c_e*L*cos(phi)];
     
LfLfh = [-(c_d^2*b*sin(phi)+c_d^2*L*cos(phi))*thetaD_d^2 + (c_e^2*b*sin(phi)-c_e^2*L*cos(phi))*thetaE_d^2 + 2*c_d*c_e*L*cos(phi)*thetaD_d*thetaE_d;
          (c_d^2*b*cos(phi)-c_d^2*L*sin(phi))*thetaD_d^2 - (c_e^2*b*cos(phi)+c_e^2*L*sin(phi))*thetaE_d^2 + 2*c_d*c_e*L*sin(phi)*thetaD_d*thetaE_d];
   
%--------------------------------------------------------------------------
micro = LgLfh^-1*(u-LfLfh);

== matlab function modelo_matematico/Saída/Saídas ==
  data: xr output; yr output; xr_d output; yr_d output; cte input; x input
function [xr, yr, xr_d, yr_d] = fcn(cte, x)
%#codegen
% Parametros de simulação--------------------------------------------------

b   = cte(1,1);
c_d = cte(1,2);
c_e = cte(1,3);
L   = cte(1,4);

%--------------------------------------------------------------------------
xo       = x(1,1);
yo       = x(2,1);
thetaD_d = x(5,1);
thetaE_d = x(6,1);
phi      = c_d*x(3,1)-c_e*x(4,1);

%--------------------------------------------------------------------------
Lfh = [c_d*b*cos(phi)*thetaD_d+c_e*b*cos(phi)*thetaE_d-c_d*L*sin(phi)*thetaD_d+c_e*L*sin(phi)*thetaE_d;
       c_d*b*sin(phi)*thetaD_d+c_e*b*sin(phi)*thetaE_d+c_d*L*cos(phi)*thetaD_d-c_e*L*cos(phi)*thetaE_d];

xr_d = Lfh(1,1);
yr_d = Lfh(2,1);

xr = xo + L*cos(phi);
yr = yo + L*sin(phi);

== matlab function modelo_matematico/Cancelamento da dinâmica/Transformação da Entrada ==
  data: cte input; micro input; x input; tauD output; tauE output
function [tauD, tauE] = fcn(cte, micro, x)
%#codegen
% Parametros de simulação--------------------------------------------------
% eta = η;

b   = cte(1,1);
r_d = cte(1,2);
r_e = cte(1,3);
c_d = cte(1,4);
c_e = cte(1,5);
Ir  = cte(1,6);
m   = cte(1,7);
I   = cte(1,8);

%--------------------------------------------------------------------------
thetaD_d = x(5,1);
thetaE_d = x(6,1);
phi      = c_d*x(3,1)-c_e*x(4,1);

%--------------------------------------------------------------------------
S = [ c_d*b*cos(phi) , c_e*b*cos(phi) ;
      c_d*b*sin(phi) , c_e*b*sin(phi) ;
            1        ,       0        ;
            0        ,       1        ];
               
S_d = [ -(r_d^2/4*b)*sin(phi)*thetaD_d + (r_d*r_e/4*b)*sin(phi)*thetaE_d , -(r_d*r_e/4*b)*sin(phi)*thetaD_d + (r_e^2/4*b)*sin(phi)*thetaE_d;
         (r_d^2/4*b)*cos(phi)*thetaD_d - (r_d*r_e/4*b)*cos(phi)*thetaE_d ,  (r_d*r_e/4*b)*cos(phi)*thetaD_d - (r_e^2/4*b)*cos(phi)*thetaE_d;
                                       0                                 ,                                  0                              ;
                                       0                                 ,                                  0                              ];
                        
M = [ m , 0 ,       0    ,       0    ;
      0 , m ,       0    ,       0    ;
      0 , 0 , Ir+I*c_d^2 ,   -I*c_e^2 ;
      0 , 0 ,   -I*c_d^2 , Ir+I*c_e^2 ];
            
eta = [thetaD_d;
       thetaE_d];
   
% Cálculo de tau-----------------------------------------------------------

tau  = (S'*M*S_d*eta) + S'*M*S*micro;
tauD = tau(1,1);
tauE = tau(2,1);
